simulink model "init_sim"  (R2018b)
settings: Solver=VariableStepAuto  StartTime=0.0  StopTime=endtime  RelTol=1e-3
libraries: simulink x1
settings Model: Creator=Tarunbir Singh  LastModifiedBy=Tarunbir Singh

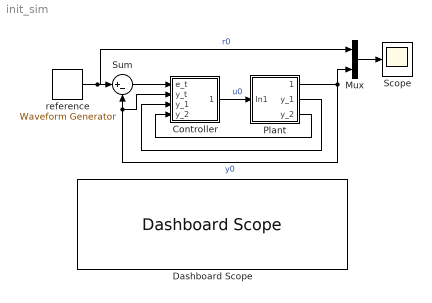
== system init_sim ==
  "Controller " : Subsystem
  Dashboard Scope : DashboardScope  WebBlockId=123
  Mux : Mux  Inputs=2
  "Plant " : Subsystem
  Scope : Scope
  Sum : Sum  Inputs=|+-
  "reference " : simulink/Sources/Waveform Generator  OutMin=[]  OutMax=[]  OutDataTypeStr=double  SelectedSignal=1  Signals=step(0,0,0.5) + step(50,0,0.5) + step(100,0,1) + step(150,0,-0.5)  BlockNames=MultiportSwitch_c8cc2258f1b84cf  SampleTime=1
      settings: SourceProductName=Simulink
  wires:
  "Plant "/1(Out1) -> Mux/2, "Controller "/2(y_t), Sum/2  "y0"
  Mux/1 -> Scope/1
  "reference "/1 -> Mux/1, Sum/1  "r0"
  Sum/1 -> "Controller "/1("e_t ")
  "Controller "/1(Out1) -> "Plant "/1(In1)  "u0"
  "Plant "/3("y_2 ") -> "Controller "/4(y_2)
  "Plant "/2(y_1) -> "Controller "/3("y_1 ")

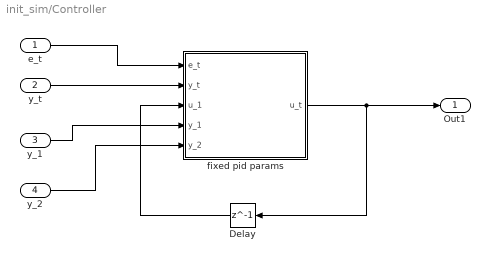
== system init_sim/Controller  ==
  "e_t " : Inport
  y_t : Inport  Port=2
  "y_1 " : Inport  Port=3
  y_2 : Inport  Port=4
  Delay : Delay  DelayLength=1  SampleTime=1
  fixed pid params : MATLAB Function  TreatAsAtomicUnit=on
  Out1 : Outport
  wires:
  "e_t "/1 -> fixed pid params/1(e_t)
  fixed pid params/1(u_t) -> Delay/1, Out1/1
  Delay/1 -> fixed pid params/3(u_1)
  "y_1 "/1 -> fixed pid params/4(y_1)
  y_2/1 -> fixed pid params/5(y_2)
  y_t/1 -> fixed pid params/2(y_t)

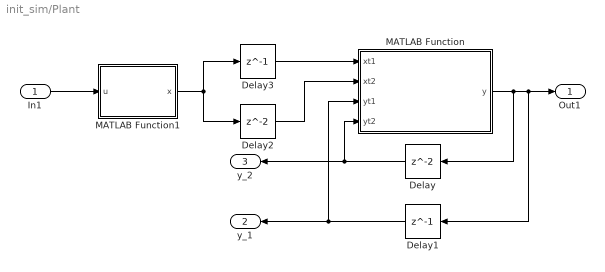
== system init_sim/Plant  ==
  In1 : Inport
  Delay : Delay  InitialCondition=0  SampleTime=1
  Delay1 : Delay  DelayLength=1  InitialCondition=0  SampleTime=1
  Delay2 : Delay  InitialCondition=0  SampleTime=1
  Delay3 : Delay  DelayLength=1  InitialCondition=0  SampleTime=1
  MATLAB Function : MATLAB Function  TreatAsAtomicUnit=on
  MATLAB Function1 : MATLAB Function  TreatAsAtomicUnit=on
  Out1 : Outport
  y_1 : Outport  Port=2
  "y_2 " : Outport  Port=3
  wires:
  In1/1 -> MATLAB Function1/1(u)
  MATLAB Function/1(y) -> Delay/1, Delay1/1, Out1/1
  Delay/1 -> "y_2 "/1, MATLAB Function/4(yt2)
  Delay1/1 -> y_1/1, MATLAB Function/3(yt1)
  MATLAB Function1/1(x) -> Delay3/1, Delay2/1
  Delay2/1 -> MATLAB Function/2(xt2)
  Delay3/1 -> MATLAB Function/1(xt1)

== matlab function init_sim/Plant /MATLAB Function1 ==
  data: u input; x output
function x = fcn(u)

x = 1.5*u - 1.5*u^2 + 0.5*u^3;

== matlab function init_sim/Plant /MATLAB Function ==
  data: xt1 input; y output; xt2 input; yt1 input; yt2 input
function y = fcn(xt1,xt2,yt1,yt2)

y = 0.6*yt1 - 0.1*yt2 + 1.2*xt1 - 0.1*xt2;

== matlab function init_sim/Controller /fixed pid params ==
  data: e_t input; u_t output; y_t input; u_1 input; y_1 input; y_2 input; K parameter
function u_t = fcn(e_t, y_t, u_1, y_1, y_2, K)

u_t = u_1 + K(2)*(e_t) - K(1)*(y_t - y_1) - K(3)*(y_t - 2*y_1 + y_2);
